simulink model "QPSK_Transmit_v14"  (R2012b)
settings: Solver=FixedStepDiscrete  SolverMode=SingleTasking  StartTime=0.0  StopTime=4000  FixedStep=1  RelTol=1e-3
libraries: simulink x23
settings Model: FPTRunName=FPA_Reference  Creator=Carl  LastModifiedBy=Girish
settings DataIOCC: SignalLogging=off
settings OptimizationCC: BlockReduction=off  ConditionallyExecuteInputs=off  InlineParams=on
settings DebuggingCC: AlgebraicLoopMsg=error
settings HardwareCC: ProdHWDeviceType=ASIC/FPGA->ASIC/FPGA  ProdEqTarget=off

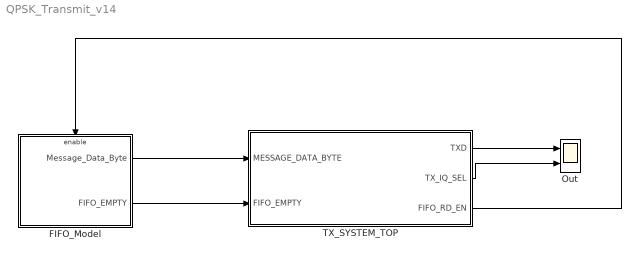
== system QPSK_Transmit_v14 ==
  FIFO_Model : Subsystem
  Out : Scope  NumInputPorts=2
      settings: YMin=-5~-5  YMax=5~5  SaveName=ScopeData7
  TX_SYSTEM_TOP : Subsystem
  wires:
  FIFO_Model/1(Message_Data_Byte) -> TX_SYSTEM_TOP/1(MESSAGE_DATA_BYTE)
  FIFO_Model/2(FIFO_EMPTY) -> TX_SYSTEM_TOP/2(FIFO_EMPTY)
  TX_SYSTEM_TOP/3(FIFO_RD_EN) -> FIFO_Model/Enable
  TX_SYSTEM_TOP/1(TXD) -> Out/1
  TX_SYSTEM_TOP/2(TX_IQ_SEL) -> Out/2

== system QPSK_Transmit_v14/FIFO_Model ==
  Enable : EnablePort
  Compare To Constant5 : simulink/Logic and Bit Operations/Compare To Constant  relop===  const=17  OutDataTypeStr=boolean  ZeroCross=off
  Delay : Delay  DelayLength=1  InitialCondition=0
  Message_Data_LUT : LookupNDDirect  NumberOfTableDimensions=1  Table="[12        0        0        1        104        101        108        108        111        32        119        111        114        108        100        33        198        228]"  DiagnosticForOutOfRangeInput=Error  TableDataTypeStr=uint8
  Scope : Scope
  reset_counter : Subsystem  AncestorBlock=hdldemolib/HDL Streaming FFT/enable_counter
  Message_Data_Byte : Outport
  FIFO_EMPTY : Outport  Port=2
  wires:
  Message_Data_LUT/1 -> Message_Data_Byte/1
  reset_counter/1(sclock) -> Compare To Constant5/1, Scope/1, Message_Data_LUT/1
  Compare To Constant5/1 -> Delay/1, FIFO_EMPTY/1
  Delay/1 -> reset_counter/1(reset)

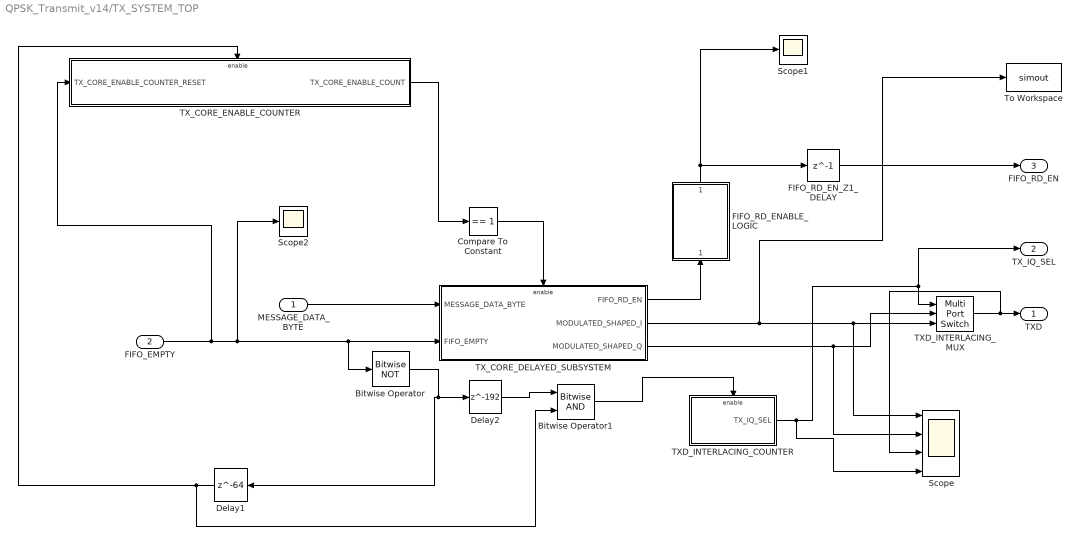
== system QPSK_Transmit_v14/TX_SYSTEM_TOP ==
  MESSAGE_DATA_BYTE : Inport
  FIFO_EMPTY : Inport  Port=2
  Bitwise Operator : simulink/Logic and Bit Operations/Bitwise Operator  logicop=NOT  UseBitMask=off  BitMask=bin2dec('11011001')  BitMaskRealWorld=Stored Integer
  Bitwise Operator1 : simulink/Logic and Bit Operations/Bitwise Operator  logicop=AND  UseBitMask=off  NumInputPorts=2  BitMask=bin2dec('11011001')  BitMaskRealWorld=Stored Integer
  Compare To Constant : simulink/Logic and Bit Operations/Compare To Constant  relop===  const=1  OutDataTypeStr=boolean
  Delay1 : Delay  DelayLength=64  InitialCondition=0
  Delay2 : Delay  DelayLength=192  InitialCondition=0
  FIFO_RD_ENABLE_LOGIC : Subsystem  AncestorBlock=hdldemolib/HDL Streaming FFT/enable_counter
  FIFO_RD_EN_Z1_DELAY : Delay  DelayLength=1  InitialCondition=0
  Scope : Scope  NumInputPorts=4
      settings: YMin=-5~-5~-5~-5  YMax=5~5~5~5
  Scope1 : Scope
      settings: SaveName=ScopeData8
  Scope2 : Scope
      settings: SaveName=ScopeData9
  "TXD_INTERLACING_COUNTER " : Subsystem
  TXD_INTERLACING_MUX : MultiPortSwitch  DataPortOrder=Zero-based contiguous  Inputs=2  zeroidx=on
  TX_CORE_DELAYED_SUBSYSTEM : Subsystem
  TX_CORE_ENABLE_COUNTER : Subsystem  AncestorBlock=hdldemolib/HDL Streaming FFT/enable_counter
  To Workspace : ToWorkspace  VariableName=simout  SampleTime=-1
  TXD : Outport
  TX_IQ_SEL : Outport  Port=2
  FIFO_RD_EN : Outport  Port=3
  wires:
  FIFO_RD_EN_Z1_DELAY/1 -> FIFO_RD_EN/1
  MESSAGE_DATA_BYTE/1 -> TX_CORE_DELAYED_SUBSYSTEM/1(MESSAGE_DATA_BYTE)
  TXD_INTERLACING_MUX/1 -> Scope/3, TXD/1
  TX_CORE_DELAYED_SUBSYSTEM/3(MODULATED_SHAPED_Q) -> Scope/2, TXD_INTERLACING_MUX/2
  TX_CORE_DELAYED_SUBSYSTEM/2(MODULATED_SHAPED_I) -> To Workspace/1, Scope/1, TXD_INTERLACING_MUX/3
  TX_CORE_ENABLE_COUNTER/1(TX_CORE_ENABLE_COUNT) -> Compare To Constant/1
  "TXD_INTERLACING_COUNTER "/1("TX_IQ_SEL ") -> Scope/4, TX_IQ_SEL/1, TXD_INTERLACING_MUX/1
  FIFO_EMPTY/1 -> TX_CORE_ENABLE_COUNTER/1(TX_CORE_ENABLE_COUNTER_RESET), Scope2/1, TX_CORE_DELAYED_SUBSYSTEM/2(FIFO_EMPTY), Bitwise Operator/1
  Compare To Constant/1 -> TX_CORE_DELAYED_SUBSYSTEM/Enable
  TX_CORE_DELAYED_SUBSYSTEM/1(FIFO_RD_EN) -> FIFO_RD_ENABLE_LOGIC/1(FIFO_RD_ENABLE_LOGIC_INPUT)
  FIFO_RD_ENABLE_LOGIC/1(FIFO_RD_ENABLE_LOGIC_OUTPUT) -> Scope1/1, FIFO_RD_EN_Z1_DELAY/1
  Bitwise Operator/1 -> Delay2/1, Delay1/1
  Delay1/1 -> Bitwise Operator1/2, TX_CORE_ENABLE_COUNTER/Enable
  Delay2/1 -> Bitwise Operator1/1
  Bitwise Operator1/1 -> "TXD_INTERLACING_COUNTER "/Enable

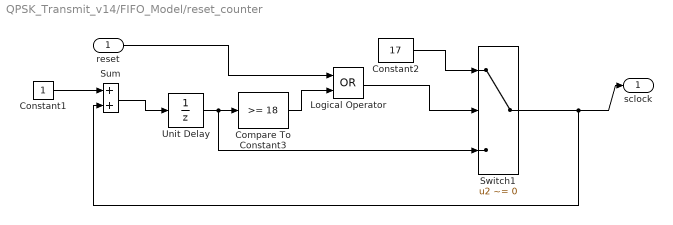
== system QPSK_Transmit_v14/FIFO_Model/reset_counter ==
  reset : Inport
  Compare To Constant3 : simulink/Logic and Bit Operations/Compare To Constant  relop=>=  const=18  OutDataTypeStr=boolean  ZeroCross=off
  Constant1 : Constant  OutDataTypeStr=int8  SampleTime=-1
  Constant2 : Constant  Value=17  OutDataTypeStr=int8  SampleTime=-1
  Logical Operator : Logic  Operator=OR  AllPortsSameDT=off  OutDataTypeStr=boolean
  Sum : Sum  AccumDataTypeStr=int8  RndMeth=Nearest  SaturateOnIntegerOverflow=on
  Switch1 : Switch  Criteria=u2 ~= 0
  Unit Delay : UnitDelay  SampleTime=-1
  sclock : Outport
  wires:
  Switch1/1 -> Sum/2, sclock/1
  Unit Delay/1 -> Compare To Constant3/1, Switch1/3
  Constant2/1 -> Switch1/1
  Sum/1 -> Unit Delay/1
  Constant1/1 -> Sum/1
  Compare To Constant3/1 -> Logical Operator/2
  reset/1 -> Logical Operator/1
  Logical Operator/1 -> Switch1/2

== system QPSK_Transmit_v14/TX_SYSTEM_TOP/FIFO_RD_ENABLE_LOGIC ==
  FIFO_RD_ENABLE_LOGIC_INPUT : Inport
  Bitwise Operator : simulink/Logic and Bit Operations/Bitwise Operator  logicop=AND  UseBitMask=off  NumInputPorts=2  BitMask=bin2dec('11011001')  BitMaskRealWorld=Stored Integer
  Compare To Constant : simulink/Logic and Bit Operations/Compare To Constant  relop===  const=1  OutDataTypeStr=boolean
  Compare To Constant1 : simulink/Logic and Bit Operations/Compare To Constant  relop===  const=0  OutDataTypeStr=boolean
  Delay : Delay  DelayLength=1  InitialCondition=0
  FIFO_RD_ENABLE_LOGIC_OUTPUT : Outport  InitialOutput=0
  wires:
  FIFO_RD_ENABLE_LOGIC_INPUT/1 -> Compare To Constant/1, Delay/1
  Delay/1 -> Compare To Constant1/1
  Compare To Constant/1 -> Bitwise Operator/1
  Compare To Constant1/1 -> Bitwise Operator/2
  Bitwise Operator/1 -> FIFO_RD_ENABLE_LOGIC_OUTPUT/1

== system QPSK_Transmit_v14/TX_SYSTEM_TOP/TXD_INTERLACING_COUNTER  ==
  Enable : EnablePort
  Counter Free-Running : simulink/Sources/Counter Free-Running  NumBits=1  tsamp=-1
  "TX_IQ_SEL " : Outport  InitialOutput=0
  wires:
  Counter Free-Running/1 -> "TX_IQ_SEL "/1

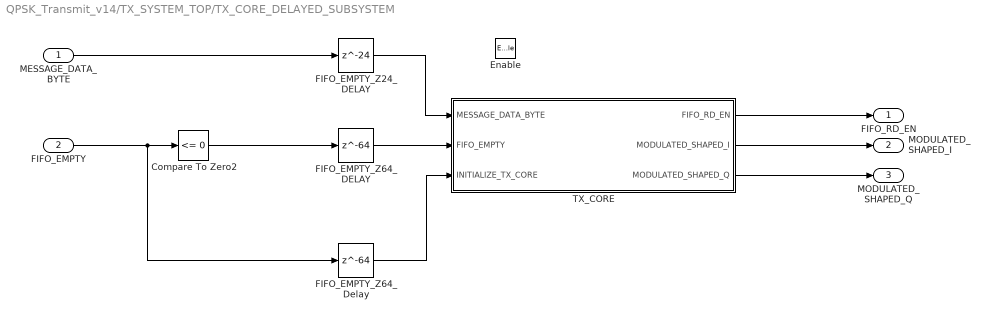
== system QPSK_Transmit_v14/TX_SYSTEM_TOP/TX_CORE_DELAYED_SUBSYSTEM ==
  MESSAGE_DATA_BYTE : Inport
  FIFO_EMPTY : Inport  Port=2
  Enable : EnablePort
  Compare To Zero2 : simulink/Logic and Bit Operations/Compare To Zero  relop=<=  OutDataTypeStr=boolean
  FIFO_EMPTY_Z24_DELAY : Delay  DelayLength=24  InitialCondition=0
  FIFO_EMPTY_Z64_DELAY : Delay  DelayLength=64  InitialCondition=0
  FIFO_EMPTY_Z64_Delay : Delay  DelayLength=64  InitialCondition=0
  TX_CORE : Subsystem
  FIFO_RD_EN : Outport  InitialOutput=0
  MODULATED_SHAPED_I : Outport  Port=2  InitialOutput=0
  MODULATED_SHAPED_Q : Outport  Port=3  InitialOutput=0
  wires:
  MESSAGE_DATA_BYTE/1 -> FIFO_EMPTY_Z24_DELAY/1
  FIFO_EMPTY_Z64_Delay/1 -> TX_CORE/3(INITIALIZE_TX_CORE)
  FIFO_EMPTY_Z64_DELAY/1 -> TX_CORE/2(FIFO_EMPTY)
  Compare To Zero2/1 -> FIFO_EMPTY_Z64_DELAY/1
  FIFO_EMPTY_Z24_DELAY/1 -> TX_CORE/1(MESSAGE_DATA_BYTE)
  TX_CORE/2(MODULATED_SHAPED_I) -> MODULATED_SHAPED_I/1
  TX_CORE/3(MODULATED_SHAPED_Q) -> MODULATED_SHAPED_Q/1
  FIFO_EMPTY/1 -> FIFO_EMPTY_Z64_Delay/1, Compare To Zero2/1
  TX_CORE/1(FIFO_RD_EN) -> FIFO_RD_EN/1

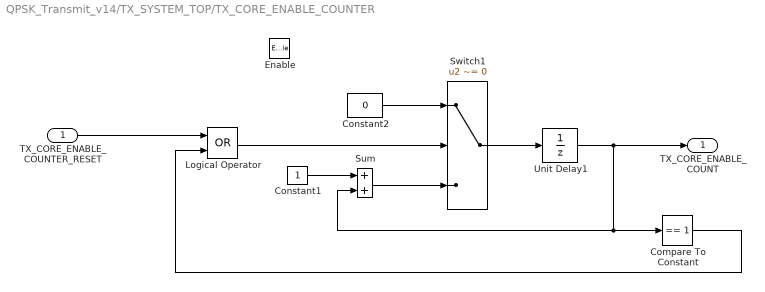
== system QPSK_Transmit_v14/TX_SYSTEM_TOP/TX_CORE_ENABLE_COUNTER ==
  TX_CORE_ENABLE_COUNTER_RESET : Inport
  Enable : EnablePort
  Compare To Constant : simulink/Logic and Bit Operations/Compare To Constant  relop===  const=1  OutDataTypeStr=boolean
  Constant1 : Constant  OutDataTypeStr=uint32
  Constant2 : Constant  Value=0  OutDataTypeStr=uint32
  Logical Operator : Logic  Operator=OR  AllPortsSameDT=off  OutDataTypeStr=boolean
  Sum : Sum  OutDataTypeStr=uint32  RndMeth=Nearest  SaturateOnIntegerOverflow=on
  Switch1 : Switch  Criteria=u2 ~= 0
  Unit Delay1 : UnitDelay  SampleTime=-1
  TX_CORE_ENABLE_COUNT : Outport  InitialOutput=0
  wires:
  Switch1/1 -> Unit Delay1/1
  Sum/1 -> Switch1/3
  Constant2/1 -> Switch1/1
  Constant1/1 -> Sum/1
  Logical Operator/1 -> Switch1/2
  Unit Delay1/1 -> TX_CORE_ENABLE_COUNT/1, Sum/2, Compare To Constant/1
  TX_CORE_ENABLE_COUNTER_RESET/1 -> Logical Operator/1
  Compare To Constant/1 -> Logical Operator/2

== system QPSK_Transmit_v14/TX_SYSTEM_TOP/TX_CORE_DELAYED_SUBSYSTEM/TX_CORE ==
  MESSAGE_DATA_BYTE : Inport
  FIFO_EMPTY : Inport  Port=2
  INITIALIZE_TX_CORE : Inport  Port=3
  GEN_MOD_SHAPED_TX_DATA_PACKET : Subsystem
  FIFO_RD_EN : Outport
  MODULATED_SHAPED_I : Outport  Port=2
  MODULATED_SHAPED_Q : Outport  Port=3
  wires:
  INITIALIZE_TX_CORE/1 -> GEN_MOD_SHAPED_TX_DATA_PACKET/2(INITIALIZE_TX_CORE)
  GEN_MOD_SHAPED_TX_DATA_PACKET/2(MODULATED_SHAPED_I) -> MODULATED_SHAPED_I/1
  GEN_MOD_SHAPED_TX_DATA_PACKET/1(FIFO_RD_EN) -> FIFO_RD_EN/1
  MESSAGE_DATA_BYTE/1 -> GEN_MOD_SHAPED_TX_DATA_PACKET/1(MESSAGE_DATA_BYTE)
  GEN_MOD_SHAPED_TX_DATA_PACKET/3(MODULATED_SHAPED_Q) -> MODULATED_SHAPED_Q/1
  FIFO_EMPTY/1 -> GEN_MOD_SHAPED_TX_DATA_PACKET/Enable

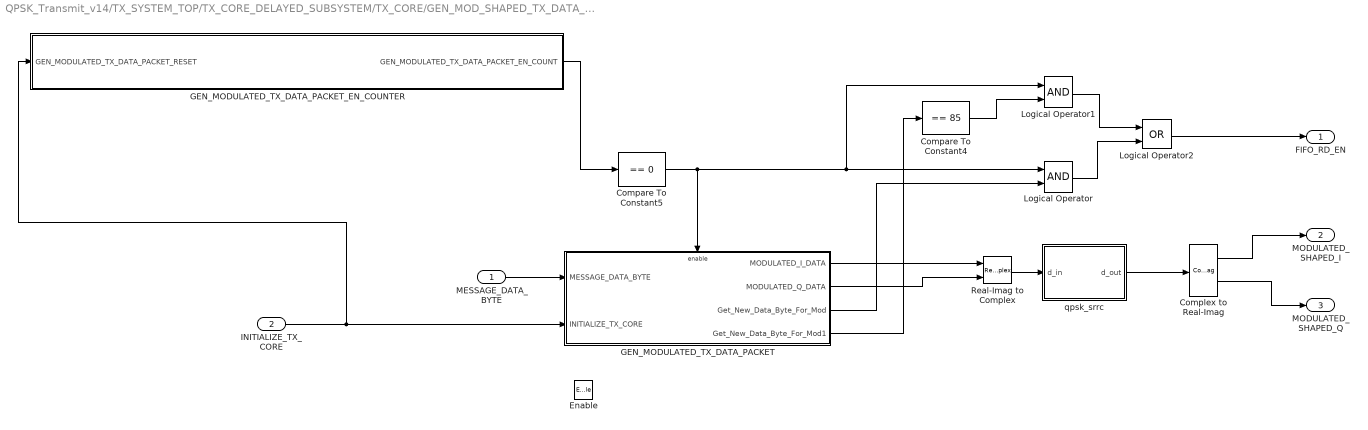
== system QPSK_Transmit_v14/TX_SYSTEM_TOP/TX_CORE_DELAYED_SUBSYSTEM/TX_CORE/GEN_MOD_SHAPED_TX_DATA_PACKET ==
  MESSAGE_DATA_BYTE : Inport
  INITIALIZE_TX_CORE : Inport  Port=2
  Enable : EnablePort
  Compare To Constant4 : simulink/Logic and Bit Operations/Compare To Constant  relop===  const=85  OutDataTypeStr=boolean  ZeroCross=off
  Compare To Constant5 : simulink/Logic and Bit Operations/Compare To Constant  relop===  const=0  OutDataTypeStr=boolean  ZeroCross=off
  Complex to Real-Imag : ComplexToRealImag
  GEN_MODULATED_TX_DATA_PACKET : Subsystem
  GEN_MODULATED_TX_DATA_PACKET_EN_COUNTER : Subsystem  AncestorBlock=hdldemolib/HDL Streaming FFT/enable_counter
  Logical Operator : Logic  AllPortsSameDT=off  OutDataTypeStr=boolean
  Logical Operator1 : Logic  AllPortsSameDT=off  OutDataTypeStr=boolean
  Logical Operator2 : Logic  Operator=OR  AllPortsSameDT=off  OutDataTypeStr=boolean
  Real-Imag to Complex : RealImagToComplex
  qpsk_srrc : MATLAB Function  TreatAsAtomicUnit=on
  FIFO_RD_EN : Outport  InitialOutput=0
  MODULATED_SHAPED_I : Outport  Port=2  InitialOutput=0
  MODULATED_SHAPED_Q : Outport  Port=3  InitialOutput=0
  wires:
  Complex to Real-Imag/1 -> MODULATED_SHAPED_I/1
  Complex to Real-Imag/2 -> MODULATED_SHAPED_Q/1
  GEN_MODULATED_TX_DATA_PACKET/1(MODULATED_I_DATA) -> Real-Imag to Complex/1
  GEN_MODULATED_TX_DATA_PACKET/2(MODULATED_Q_DATA) -> Real-Imag to Complex/2
  MESSAGE_DATA_BYTE/1 -> GEN_MODULATED_TX_DATA_PACKET/1(MESSAGE_DATA_BYTE)
  GEN_MODULATED_TX_DATA_PACKET/3(Get_New_Data_Byte_For_Mod) -> Logical Operator/2
  Compare To Constant5/1 -> Logical Operator1/1, Logical Operator/1, GEN_MODULATED_TX_DATA_PACKET/Enable
  Compare To Constant4/1 -> Logical Operator1/2
  GEN_MODULATED_TX_DATA_PACKET/4(Get_New_Data_Byte_For_Mod1) -> Compare To Constant4/1
  Logical Operator/1 -> Logical Operator2/2
  Logical Operator1/1 -> Logical Operator2/1
  Logical Operator2/1 -> FIFO_RD_EN/1
  GEN_MODULATED_TX_DATA_PACKET_EN_COUNTER/1(GEN_MODULATED_TX_DATA_PACKET_EN_COUNT) -> Compare To Constant5/1
  INITIALIZE_TX_CORE/1 -> GEN_MODULATED_TX_DATA_PACKET_EN_COUNTER/1(GEN_MODULATED_TX_DATA_PACKET_RESET), GEN_MODULATED_TX_DATA_PACKET/2(INITIALIZE_TX_CORE)
  Real-Imag to Complex/1 -> qpsk_srrc/1(d_in)
  qpsk_srrc/1(d_out) -> Complex to Real-Imag/1

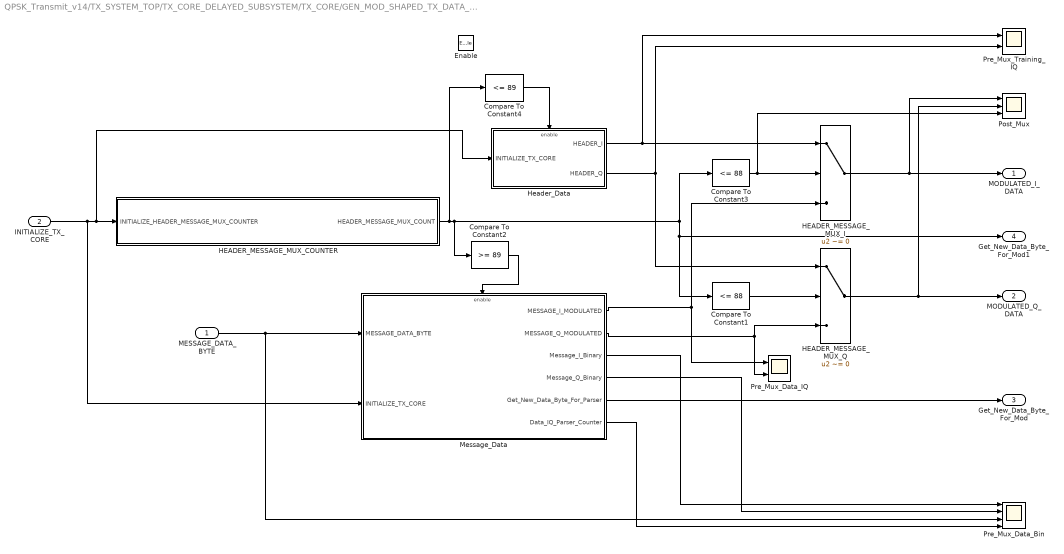
== system QPSK_Transmit_v14/TX_SYSTEM_TOP/TX_CORE_DELAYED_SUBSYSTEM/TX_CORE/GEN_MOD_SHAPED_TX_DATA_PACKET/GEN_MODULATED_TX_DATA_PACKET ==
  MESSAGE_DATA_BYTE : Inport
  INITIALIZE_TX_CORE : Inport  Port=2
  Enable : EnablePort
  Compare To Constant1 : simulink/Logic and Bit Operations/Compare To Constant  relop=<=  const=88  OutDataTypeStr=boolean  ZeroCross=off
  Compare To Constant2 : simulink/Logic and Bit Operations/Compare To Constant  relop=>=  const=89  OutDataTypeStr=boolean  ZeroCross=off
  Compare To Constant3 : simulink/Logic and Bit Operations/Compare To Constant  relop=<=  const=88  OutDataTypeStr=boolean  ZeroCross=off
  Compare To Constant4 : simulink/Logic and Bit Operations/Compare To Constant  relop=<=  const=89  OutDataTypeStr=boolean  ZeroCross=off
  HEADER_MESSAGE_MUX_COUNTER : Subsystem  AncestorBlock=hdldemolib/HDL Streaming FFT/enable_counter
  HEADER_MESSAGE_MUX_I : Switch  Criteria=u2 ~= 0  OutDataTypeStr=int8
  HEADER_MESSAGE_MUX_Q : Switch  Criteria=u2 ~= 0  OutDataTypeStr=int8
  Header_Data : Subsystem
  Message_Data : Subsystem
  Post_Mux : Scope  NumInputPorts=3
      settings: YMin=-5~-5~-5  YMax=5~5~5  SaveName=ScopeData2
  Pre_Mux_Data_Bin : Scope  NumInputPorts=4
      settings: TimeRange=1500  YMin=-0.2~-0.2~-10~-5  YMax=1.2~1.2~265~5  SaveName=ScopeData6
  Pre_Mux_Data_IQ : Scope  NumInputPorts=2
      settings: YMin=-5~-5  YMax=5~5  SaveName=ScopeData5
  Pre_Mux_Training_IQ : Scope  NumInputPorts=2
      settings: YMin=-5~-5  YMax=5~5  SaveName=ScopeData4
  MODULATED_I_DATA : Outport  InitialOutput=0
  MODULATED_Q_DATA : Outport  Port=2  InitialOutput=0
  Get_New_Data_Byte_For_Mod : Outport  Port=3  InitialOutput=0
  Get_New_Data_Byte_For_Mod1 : Outport  Port=4  InitialOutput=0
  wires:
  HEADER_MESSAGE_MUX_COUNTER/1(HEADER_MESSAGE_MUX_COUNT) -> Compare To Constant4/1, Compare To Constant3/1, Get_New_Data_Byte_For_Mod1/1, Compare To Constant1/1, Compare To Constant2/1
  HEADER_MESSAGE_MUX_I/1 -> MODULATED_I_DATA/1, Post_Mux/1
  Header_Data/1(HEADER_I) -> HEADER_MESSAGE_MUX_I/1, Pre_Mux_Training_IQ/1
  Compare To Constant1/1 -> HEADER_MESSAGE_MUX_Q/2
  HEADER_MESSAGE_MUX_Q/1 -> Post_Mux/2, MODULATED_Q_DATA/1
  Header_Data/2(HEADER_Q) -> HEADER_MESSAGE_MUX_Q/1, Pre_Mux_Training_IQ/2
  Message_Data/2(MESSAGE_Q_MODULATED) -> Pre_Mux_Data_IQ/2, HEADER_MESSAGE_MUX_Q/3
  Message_Data/1(MESSAGE_I_MODULATED) -> Pre_Mux_Data_IQ/1, HEADER_MESSAGE_MUX_I/3
  Message_Data/3(Message_I_Binary) -> Pre_Mux_Data_Bin/1
  Message_Data/4(Message_Q_Binary) -> Pre_Mux_Data_Bin/2
  Compare To Constant2/1 -> Message_Data/Enable
  Compare To Constant4/1 -> Header_Data/Enable
  MESSAGE_DATA_BYTE/1 -> Message_Data/1(MESSAGE_DATA_BYTE), Pre_Mux_Data_Bin/3
  Compare To Constant3/1 -> Post_Mux/3, HEADER_MESSAGE_MUX_I/2
  Message_Data/5(Get_New_Data_Byte_For_Parser) -> Get_New_Data_Byte_For_Mod/1
  Message_Data/6(Data_IQ_Parser_Counter) -> Pre_Mux_Data_Bin/4
  INITIALIZE_TX_CORE/1 -> HEADER_MESSAGE_MUX_COUNTER/1(INITIALIZE_HEADER_MESSAGE_MUX_COUNTER), Header_Data/1(INITIALIZE_TX_CORE), Message_Data/2(INITIALIZE_TX_CORE)

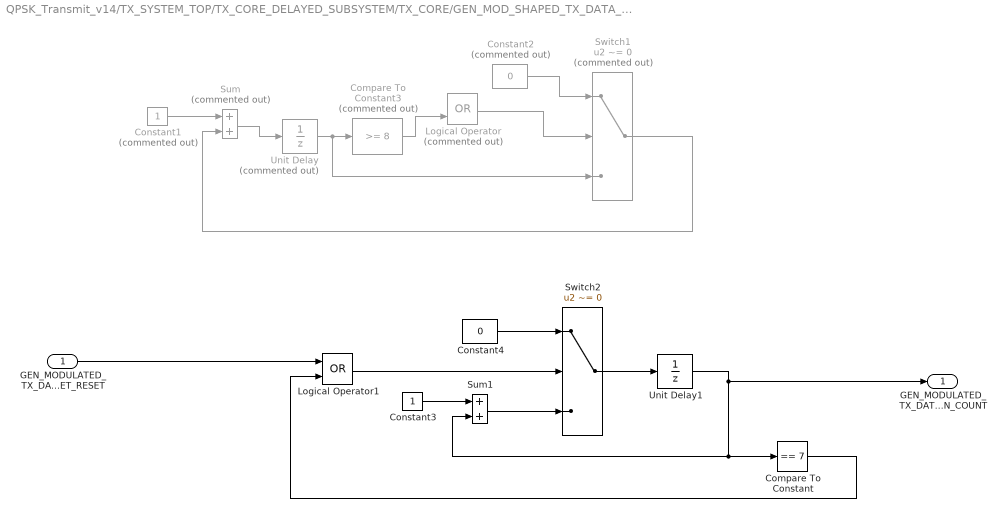
== system QPSK_Transmit_v14/TX_SYSTEM_TOP/TX_CORE_DELAYED_SUBSYSTEM/TX_CORE/GEN_MOD_SHAPED_TX_DATA_PACKET/GEN_MODULATED_TX_DATA_PACKET_EN_COUNTER ==
  GEN_MODULATED_TX_DATA_PACKET_RESET : Inport
  Compare To Constant3 : simulink/Logic and Bit Operations/Compare To Constant  Commented=on  relop=>=  const=8  OutDataTypeStr=boolean  ZeroCross=off
  Compare To Constant : simulink/Logic and Bit Operations/Compare To Constant  relop===  const=7  OutDataTypeStr=boolean
  Constant1 : Constant  Commented=on  OutDataTypeStr=int8  SampleTime=-1
  Constant2 : Constant  Commented=on  Value=0  OutDataTypeStr=int8  SampleTime=-1
  Constant3 : Constant  OutDataTypeStr=uint32
  Constant4 : Constant  Value=0  OutDataTypeStr=uint32
  Logical Operator : Logic  Commented=on  Operator=OR  AllPortsSameDT=off  OutDataTypeStr=boolean
  Logical Operator1 : Logic  Operator=OR  AllPortsSameDT=off  OutDataTypeStr=boolean
  Sum : Sum  Commented=on  OutDataTypeStr=int8  RndMeth=Nearest  SaturateOnIntegerOverflow=on
  Sum1 : Sum  OutDataTypeStr=uint32  RndMeth=Nearest  SaturateOnIntegerOverflow=on
  Switch1 : Switch  Commented=on  Criteria=u2 ~= 0
  Switch2 : Switch  Criteria=u2 ~= 0
  Unit Delay : UnitDelay  Commented=on  SampleTime=-1
  Unit Delay1 : UnitDelay  SampleTime=-1
  GEN_MODULATED_TX_DATA_PACKET_EN_COUNT : Outport  InitialOutput=0
  wires:
  Switch1/1 -> Sum/2
  Unit Delay/1 -> Compare To Constant3/1, Switch1/3
  Constant2/1 -> Switch1/1
  Sum/1 -> Unit Delay/1
  Constant1/1 -> Sum/1
  Compare To Constant3/1 -> Logical Operator/2
  Logical Operator/1 -> Switch1/2
  Switch2/1 -> Unit Delay1/1
  Sum1/1 -> Switch2/3
  Constant4/1 -> Switch2/1
  Constant3/1 -> Sum1/1
  Logical Operator1/1 -> Switch2/2
  Unit Delay1/1 -> GEN_MODULATED_TX_DATA_PACKET_EN_COUNT/1, Sum1/2, Compare To Constant/1
  Compare To Constant/1 -> Logical Operator1/2
  GEN_MODULATED_TX_DATA_PACKET_RESET/1 -> Logical Operator1/1

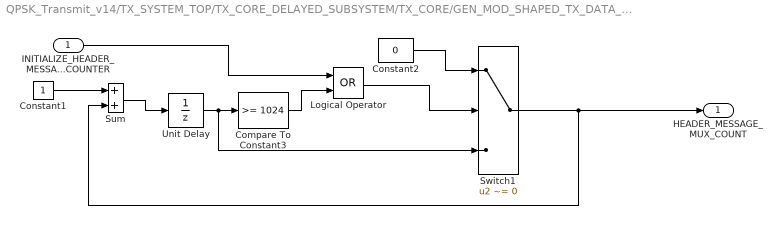
== system QPSK_Transmit_v14/TX_SYSTEM_TOP/TX_CORE_DELAYED_SUBSYSTEM/TX_CORE/GEN_MOD_SHAPED_TX_DATA_PACKET/GEN_MODULATED_TX_DATA_PACKET/HEADER_MESSAGE_MUX_COUNTER ==
  INITIALIZE_HEADER_MESSAGE_MUX_COUNTER : Inport
  Compare To Constant3 : simulink/Logic and Bit Operations/Compare To Constant  relop=>=  const=1024  OutDataTypeStr=boolean  ZeroCross=off
  Constant1 : Constant  OutDataTypeStr=int8  SampleTime=-1
  Constant2 : Constant  Value=0  OutDataTypeStr=int8  SampleTime=-1
  Logical Operator : Logic  Operator=OR  AllPortsSameDT=off  OutDataTypeStr=boolean
  Sum : Sum  OutDataTypeStr=uint32  RndMeth=Nearest  SaturateOnIntegerOverflow=on
  Switch1 : Switch  Criteria=u2 ~= 0
  Unit Delay : UnitDelay  SampleTime=-1
  HEADER_MESSAGE_MUX_COUNT : Outport
  wires:
  Switch1/1 -> Sum/2, HEADER_MESSAGE_MUX_COUNT/1
  Unit Delay/1 -> Compare To Constant3/1, Switch1/3
  Constant2/1 -> Switch1/1
  Sum/1 -> Unit Delay/1
  Constant1/1 -> Sum/1
  Compare To Constant3/1 -> Logical Operator/2
  INITIALIZE_HEADER_MESSAGE_MUX_COUNTER/1 -> Logical Operator/1
  Logical Operator/1 -> Switch1/2

== system QPSK_Transmit_v14/TX_SYSTEM_TOP/TX_CORE_DELAYED_SUBSYSTEM/TX_CORE/GEN_MOD_SHAPED_TX_DATA_PACKET/GEN_MODULATED_TX_DATA_PACKET/Header_Data ==
  INITIALIZE_TX_CORE : Inport
  Enable : EnablePort
  HEADER_SYMBOL_COUNTER : Subsystem  AncestorBlock=hdldemolib/HDL Streaming FFT/enable_counter
  Pad_Training_LUT_I : LookupNDDirect  NumberOfTableDimensions=1  Table=|  DiagnosticForOutOfRangeInput=Error  TableDataTypeStr=int8
      | [1
      | -1
      | 1
      | -1
      | 1
      | -1
      | 1
      | -1
      | 1
      | -1
      | 1
      | -1
      | 1
      | -1
      | 1
      | -1
      | 1
      | -1
      | 1
      | -1
      | 1
      | -1
      | 1
      | -1
      | 1
      | 1
      | -1
      | -1
      | 1
      | 1
      | -1
      | -1
      | 1
      | -1
      | -1
      | -1
      | -1
      | 1
      | -1
      | 1
      | 1
      | -1
      | -1
      | 1
      | 1
      | 1
      | -1
      | 1
      | 1
      | 1
      | -1
      | 1
      | -1
      | 1
      | 1
      | 1
      | -1
      | 1
      | 1
      | 1
      | 1
      | -1
      | 1
      | 1
      | -1
      | -1
      | -1
      | -1
      | 1
      | 1
      | 1
      | -1
      | -1
      | -1
      | 1
      | 1
      | 1
      | 1
      | -1
      | 1
      | 1
      | 1
      | 1
      | 1
      | -1
      | -1
      | -1
      | 1
      | 1
      | ]
  Pad_Training_LUT_Q : LookupNDDirect  NumberOfTableDimensions=1  Table=|  DiagnosticForOutOfRangeInput=Error  TableDataTypeStr=int8
      | [1
      | -1
      | 1
      | -1
      | 1
      | -1
      | 1
      | -1
      | 1
      | -1
      | 1
      | -1
      | 1
      | -1
      | 1
      | -1
      | 1
      | -1
      | 1
      | -1
      | 1
      | -1
      | 1
      | -1
      | 1
      | -1
      | 1
      | 1
      | 1
      | -1
      | -1
      | -1
      | -1
      | 1
      | 1
      | -1
      | 1
      | 1
      | -1
      | -1
      | -1
      | 1
      | -1
      | -1
      | 1
      | 1
      | 1
      | -1
      | -1
      | 1
      | 1
      | 1
      | -1
      | -1
      | -1
      | -1
      | -1
      | -1
      | 1
      | 1
      | -1
      | 1
      | -1
      | 1
      | 1
      | -1
      | -1
      | 1
      | -1
      | -1
      | 1
      | 1
      | -1
      | -1
      | -1
      | -1
      | -1
      | 1
      | 1
      | 1
      | 1
      | -1
      | -1
      | -1
      | -1
      | 1
      | -1
      | 1
      | -1
      | ]
  Training Counter : Scope  NumInputPorts=2
      settings: YMin=-5~-5  YMax=5~5  SaveName=ScopeData3
  HEADER_I : Outport  InitialOutput=0
  HEADER_Q : Outport  Port=2  InitialOutput=0
  wires:
  Pad_Training_LUT_I/1 -> HEADER_I/1
  HEADER_SYMBOL_COUNTER/1(HEADER_SYMBOL_COUNT) -> Training Counter/1, Pad_Training_LUT_I/1, Pad_Training_LUT_Q/1
  Pad_Training_LUT_Q/1 -> HEADER_Q/1
  INITIALIZE_TX_CORE/1 -> HEADER_SYMBOL_COUNTER/1(INITIALIZE_HEADER_SYMBOL_COUNTER), Training Counter/2

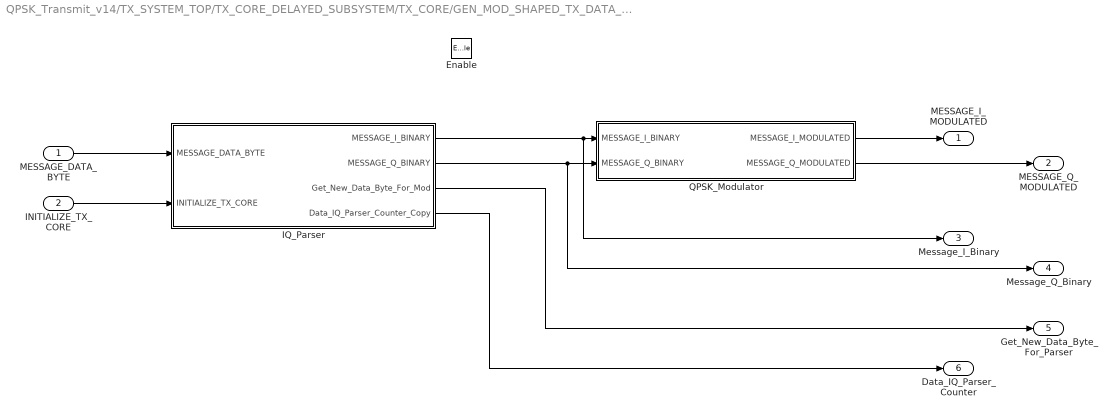
== system QPSK_Transmit_v14/TX_SYSTEM_TOP/TX_CORE_DELAYED_SUBSYSTEM/TX_CORE/GEN_MOD_SHAPED_TX_DATA_PACKET/GEN_MODULATED_TX_DATA_PACKET/Message_Data ==
  MESSAGE_DATA_BYTE : Inport
  INITIALIZE_TX_CORE : Inport  Port=2
  Enable : EnablePort
  IQ_Parser : Subsystem
  QPSK_Modulator : Subsystem
  MESSAGE_I_MODULATED : Outport  InitialOutput=0
  MESSAGE_Q_MODULATED : Outport  Port=2  InitialOutput=0
  Message_I_Binary : Outport  Port=3  InitialOutput=0
  Message_Q_Binary : Outport  Port=4  InitialOutput=0
  Get_New_Data_Byte_For_Parser : Outport  Port=5  InitialOutput=0
  Data_IQ_Parser_Counter : Outport  Port=6  InitialOutput=0
  wires:
  IQ_Parser/1(MESSAGE_I_BINARY) -> Message_I_Binary/1, QPSK_Modulator/1(MESSAGE_I_BINARY)
  IQ_Parser/2(MESSAGE_Q_BINARY) -> Message_Q_Binary/1, QPSK_Modulator/2(MESSAGE_Q_BINARY)
  QPSK_Modulator/1(MESSAGE_I_MODULATED) -> MESSAGE_I_MODULATED/1
  QPSK_Modulator/2(MESSAGE_Q_MODULATED) -> MESSAGE_Q_MODULATED/1
  MESSAGE_DATA_BYTE/1 -> IQ_Parser/1(MESSAGE_DATA_BYTE)
  IQ_Parser/3(Get_New_Data_Byte_For_Mod) -> Get_New_Data_Byte_For_Parser/1
  IQ_Parser/4(Data_IQ_Parser_Counter_Copy) -> Data_IQ_Parser_Counter/1
  INITIALIZE_TX_CORE/1 -> IQ_Parser/2(INITIALIZE_TX_CORE)

== system QPSK_Transmit_v14/TX_SYSTEM_TOP/TX_CORE_DELAYED_SUBSYSTEM/TX_CORE/GEN_MOD_SHAPED_TX_DATA_PACKET/GEN_MODULATED_TX_DATA_PACKET/Header_Data/HEADER_SYMBOL_COUNTER ==
  INITIALIZE_HEADER_SYMBOL_COUNTER : Inport
  Compare To Constant : simulink/Logic and Bit Operations/Compare To Constant  relop===  const=88  OutDataTypeStr=boolean
  Constant1 : Constant  OutDataTypeStr=uint32
  Constant2 : Constant  Value=0  OutDataTypeStr=uint32
  Logical Operator : Logic  Operator=OR  AllPortsSameDT=off  OutDataTypeStr=boolean
  Sum : Sum  OutDataTypeStr=uint32  RndMeth=Nearest  SaturateOnIntegerOverflow=on
  Switch1 : Switch  Criteria=u2 ~= 0
  Unit Delay1 : UnitDelay  SampleTime=-1
  HEADER_SYMBOL_COUNT : Outport
  wires:
  Switch1/1 -> Unit Delay1/1
  Sum/1 -> Switch1/3
  Constant2/1 -> Switch1/1
  Constant1/1 -> Sum/1
  Logical Operator/1 -> Switch1/2
  Unit Delay1/1 -> HEADER_SYMBOL_COUNT/1, Sum/2, Compare To Constant/1
  INITIALIZE_HEADER_SYMBOL_COUNTER/1 -> Logical Operator/1
  Compare To Constant/1 -> Logical Operator/2

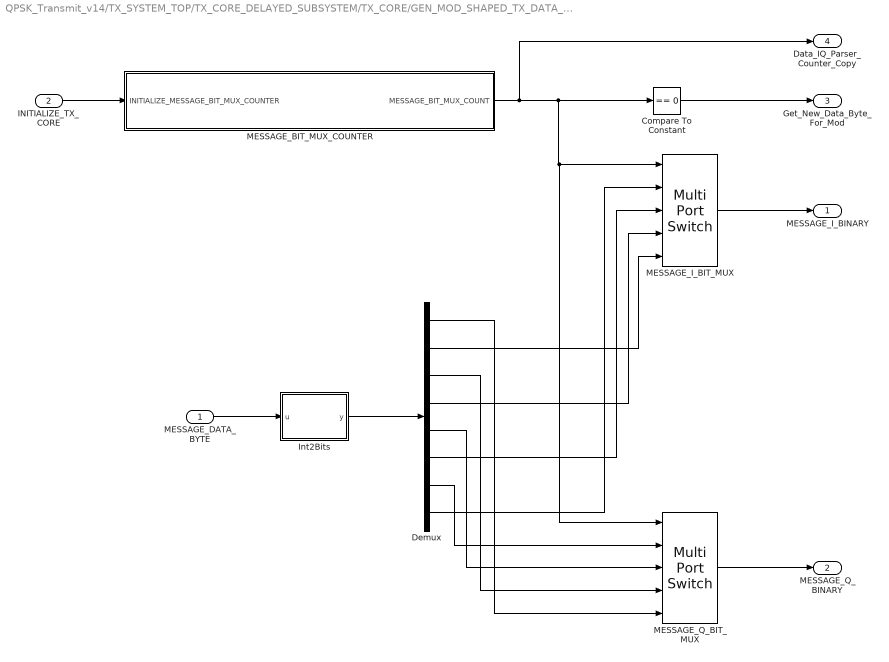
== system QPSK_Transmit_v14/TX_SYSTEM_TOP/TX_CORE_DELAYED_SUBSYSTEM/TX_CORE/GEN_MOD_SHAPED_TX_DATA_PACKET/GEN_MODULATED_TX_DATA_PACKET/Message_Data/IQ_Parser ==
  MESSAGE_DATA_BYTE : Inport
  INITIALIZE_TX_CORE : Inport  Port=2
  Compare To Constant : simulink/Logic and Bit Operations/Compare To Constant  relop===  const=0  OutDataTypeStr=boolean
  Demux : Demux  Outputs=8
  Int2Bits : MATLAB Function  TreatAsAtomicUnit=on
  MESSAGE_BIT_MUX_COUNTER : Subsystem  AncestorBlock=hdldemolib/HDL Streaming FFT/enable_counter
  MESSAGE_I_BIT_MUX : MultiPortSwitch  DataPortOrder=Zero-based contiguous  Inputs=4  zeroidx=on
  MESSAGE_Q_BIT_MUX : MultiPortSwitch  DataPortOrder=Zero-based contiguous  Inputs=4  zeroidx=on
  MESSAGE_I_BINARY : Outport
  MESSAGE_Q_BINARY : Outport  Port=2
  Get_New_Data_Byte_For_Mod : Outport  Port=3
  Data_IQ_Parser_Counter_Copy : Outport  Port=4
  wires:
  MESSAGE_Q_BIT_MUX/1 -> MESSAGE_Q_BINARY/1
  MESSAGE_BIT_MUX_COUNTER/1(MESSAGE_BIT_MUX_COUNT) -> Data_IQ_Parser_Counter_Copy/1, Compare To Constant/1, MESSAGE_I_BIT_MUX/1, MESSAGE_Q_BIT_MUX/1
  MESSAGE_I_BIT_MUX/1 -> MESSAGE_I_BINARY/1
  Demux/8 -> MESSAGE_I_BIT_MUX/2
  Demux/7 -> MESSAGE_Q_BIT_MUX/2
  Demux/6 -> MESSAGE_I_BIT_MUX/3
  Demux/5 -> MESSAGE_Q_BIT_MUX/3
  Demux/4 -> MESSAGE_I_BIT_MUX/4
  Demux/3 -> MESSAGE_Q_BIT_MUX/4
  Demux/2 -> MESSAGE_I_BIT_MUX/5
  Demux/1 -> MESSAGE_Q_BIT_MUX/5
  MESSAGE_DATA_BYTE/1 -> Int2Bits/1(u)
  Int2Bits/1(y) -> Demux/1
  Compare To Constant/1 -> Get_New_Data_Byte_For_Mod/1
  INITIALIZE_TX_CORE/1 -> MESSAGE_BIT_MUX_COUNTER/1(INITIALIZE_MESSAGE_BIT_MUX_COUNTER)

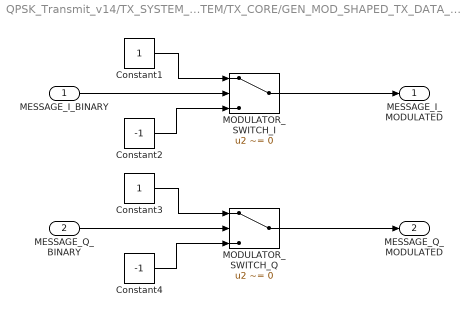
== system QPSK_Transmit_v14/TX_SYSTEM_TOP/TX_CORE_DELAYED_SUBSYSTEM/TX_CORE/GEN_MOD_SHAPED_TX_DATA_PACKET/GEN_MODULATED_TX_DATA_PACKET/Message_Data/QPSK_Modulator ==
  MESSAGE_I_BINARY : Inport
  MESSAGE_Q_BINARY : Inport  Port=2
  Constant1 : Constant  OutDataTypeStr=int8  SampleTime=-1
  Constant2 : Constant  Value=-1  OutDataTypeStr=int8  SampleTime=-1
  Constant3 : Constant  OutDataTypeStr=int8  SampleTime=-1
  Constant4 : Constant  Value=-1  OutDataTypeStr=int8  SampleTime=-1
  MODULATOR_SWITCH_I : Switch  Criteria=u2 ~= 0  RndMeth=Round
  MODULATOR_SWITCH_Q : Switch  Criteria=u2 ~= 0  RndMeth=Round
  MESSAGE_I_MODULATED : Outport
  MESSAGE_Q_MODULATED : Outport  Port=2
  wires:
  MODULATOR_SWITCH_Q/1 -> MESSAGE_Q_MODULATED/1
  Constant4/1 -> MODULATOR_SWITCH_Q/3
  Constant2/1 -> MODULATOR_SWITCH_I/3
  Constant1/1 -> MODULATOR_SWITCH_I/1
  MESSAGE_Q_BINARY/1 -> MODULATOR_SWITCH_Q/2
  Constant3/1 -> MODULATOR_SWITCH_Q/1
  MODULATOR_SWITCH_I/1 -> MESSAGE_I_MODULATED/1
  MESSAGE_I_BINARY/1 -> MODULATOR_SWITCH_I/2

== system QPSK_Transmit_v14/TX_SYSTEM_TOP/TX_CORE_DELAYED_SUBSYSTEM/TX_CORE/GEN_MOD_SHAPED_TX_DATA_PACKET/GEN_MODULATED_TX_DATA_PACKET/Message_Data/IQ_Parser/MESSAGE_BIT_MUX_COUNTER ==
  INITIALIZE_MESSAGE_BIT_MUX_COUNTER : Inport
  Compare To Constant3 : simulink/Logic and Bit Operations/Compare To Constant  relop=>=  const=4  OutDataTypeStr=boolean  ZeroCross=off
  Constant1 : Constant  OutDataTypeStr=uint32
  Constant2 : Constant  Value=0  OutDataTypeStr=uint32
  Logical Operator : Logic  Operator=OR  AllPortsSameDT=off  OutDataTypeStr=boolean
  Sum : Sum  OutDataTypeStr=uint32  RndMeth=Nearest  SaturateOnIntegerOverflow=on
  Switch1 : Switch  Criteria=u2 ~= 0
  Unit Delay : UnitDelay  SampleTime=-1
  MESSAGE_BIT_MUX_COUNT : Outport
  wires:
  Switch1/1 -> Sum/2, MESSAGE_BIT_MUX_COUNT/1
  Unit Delay/1 -> Compare To Constant3/1, Switch1/3
  Constant2/1 -> Switch1/1
  Sum/1 -> Unit Delay/1
  Constant1/1 -> Sum/1
  Compare To Constant3/1 -> Logical Operator/2
  INITIALIZE_MESSAGE_BIT_MUX_COUNTER/1 -> Logical Operator/1
  Logical Operator/1 -> Switch1/2

== matlab function QPSK_Transmit_v14/TX_SYSTEM_TOP/TX_CORE_DELAYED_SUBSYSTEM/TX_CORE/GEN_MOD_SHAPED_TX_DATA_PACKET/GEN_MODULATED_TX_DATA_PACKET/Message_Data/IQ_Parser/Int2Bits ==
  data: u input; y output
function y = fcn(u)
% Converts Integer(8bits) to a 1-D array Bits

y = bitget(u, [8:-1:1])';

== matlab function QPSK_Transmit_v14/TX_SYSTEM_TOP/TX_CORE_DELAYED_SUBSYSTEM/TX_CORE/GEN_MOD_SHAPED_TX_DATA_PACKET/qpsk_srrc ==
  data: d_in input; d_out output
function d_out  = qpsk_srrc(d_in)

fm = hdlfimath;
persistent buf
OS_RATE = 8;
f = fi(SRRC, 1, 14, 14, fm);
if isempty( buf )
    buf = fi(complex( zeros( 1,OS_RATE*2+1 ), zeros(1,OS_RATE*2+1)), 1, 3, 0, fm);
end
buf = fi([ buf( 2:end ), d_in ], 1, 3, 0, fm);
d_out = fi(buf*f, 1, 12, 11, fm);
